simulink model "SimpleEKF_2007a"  (Simulink 6.6)
settings: Solver=FixedStepDiscrete  StartTime=0.0  StopTime=300  FixedStep=0.01  RelTol=1e-3
values from neighbouring files (symbols this model uses):
  initP = diag([ 1 1 1 1e5 1e5 1 1e5 1e5 1e5 ])    [SimpleEKF_init.m.m]
undefined symbols (not defined in the file or in its folder): DiscIntNeverNeededParam, gcbh, hwbcalib_subsystem
libraries: simulink x8, dspmtrx3 x5, dspinverses x1
(part 2 of 9)

== system SimpleEKF_2007a/EKF/skewSymmetric1 ==
  skewLibIn : Inport  OutDataType=fixdt(1,16,0)  OutScaling=[]
  column1 : Selector  Tag=MBDLibrary v2007b.1  IndexOptions=Index vector (dialog)  Indices=[7 3 5]  OutputSizes=1  InputPortWidth=7  mask(Mux Selector (MBDLibrary)){InputPortWidth_mbdlib=7, Indices_mbdlib=[7 3 5]}
      mask prompts: InputPortWidth_mbdlib "Input Port Width"; Indices_mbdlib "Output Indices"
      mask help: Changes the order of the inputs.
      settings: OpenFcn=|
      | if exist('mbdlib_dialog')
      |    mbdlib_dialog(gcb,'open')
      | else
      |    open_system(gcb, 'mask')
      | end
      settings: CloseFcn=|
      | if exist('mbdlib_selector')
      |    mbdlib_selector(gcb)
      | end
      mask Help: The SELECTOR block is a MULTIPLEXED SELECTOR block, used to change the input/output order of a multiplexed data stream.
      mask Display:
      | port_label('input', 1,'[7]')
      | text(1.0,0.83333,'7', 'horizontalAlignment', 'right')
      | text(1.0,0.5,'3', 'horizontalAlignment', 'right')
      | text(1.0,0.16667,'5', 'horizontalAlignment', 'right')
  column2 : Selector  Tag=MBDLibrary v2007b.1  IndexOptions=Index vector (dialog)  Indices=[6 7 1]  OutputSizes=1  InputPortWidth=7  mask(Mux Selector (MBDLibrary)){InputPortWidth_mbdlib=7, Indices_mbdlib=[6 7 1]}
      mask prompts: InputPortWidth_mbdlib "Input Port Width"; Indices_mbdlib "Output Indices"
      mask help: Changes the order of the inputs.
      settings: OpenFcn=|
      | if exist('mbdlib_dialog')
      |    mbdlib_dialog(gcb,'open')
      | else
      |    open_system(gcb, 'mask')
      | end
      settings: CloseFcn=|
      | if exist('mbdlib_selector')
      |    mbdlib_selector(gcb)
      | end
      mask Help: The SELECTOR block is a MULTIPLEXED SELECTOR block, used to change the input/output order of a multiplexed data stream.
      mask Display:
      | port_label('input', 1,'[7]')
      | text(1.0,0.83333,'6', 'horizontalAlignment', 'right')
      | text(1.0,0.5,'7', 'horizontalAlignment', 'right')
      | text(1.0,0.16667,'1', 'horizontalAlignment', 'right')
  column3 : Selector  Tag=MBDLibrary v2007b.1  IndexOptions=Index vector (dialog)  Indices=[2 4 7]  OutputSizes=1  InputPortWidth=7  mask(Mux Selector (MBDLibrary)){InputPortWidth_mbdlib=7, Indices_mbdlib=[2 4 7]}
      mask prompts: InputPortWidth_mbdlib "Input Port Width"; Indices_mbdlib "Output Indices"
      mask help: Changes the order of the inputs.
      settings: OpenFcn=|
      | if exist('mbdlib_dialog')
      |    mbdlib_dialog(gcb,'open')
      | else
      |    open_system(gcb, 'mask')
      | end
      settings: CloseFcn=|
      | if exist('mbdlib_selector')
      |    mbdlib_selector(gcb)
      | end
      mask Help: The SELECTOR block is a MULTIPLEXED SELECTOR block, used to change the input/output order of a multiplexed data stream.
      mask Display:
      | port_label('input', 1,'[7]')
      | text(1.0,0.83333,'2', 'horizontalAlignment', 'right')
      | text(1.0,0.5,'4', 'horizontalAlignment', 'right')
      | text(1.0,0.16667,'7', 'horizontalAlignment', 'right')
  matrixConcat : Concatenate  Tag=MBDLibrary v2007b.1  NumInputs=3  Mode=Multidimensional array  ConcatenateDimension=2  mask(Matrix Concat (MBDLibrary)){concatDim=Horizontal, numInputs_mbdlib=3}
      mask prompts: concatDim "Type of Concatenate"; numInputs_mbdlib "Number of Inputs"
      mask help: Concatenate input signals of the same data type to create a contiguous output signal.
      settings: OpenFcn=|
      | if exist('mbdlib_dialog')
      |    mbdlib_dialog(gcb,'open')
      | else
      |    open_system(gcb, 'mask')
      | end
      settings: CloseFcn=|
      | if exist('mbdlib_matrixConcatenate')
      |    mbdlib_matrixConcatenate(gcb, 'mask')
      | end
      mask Help:
      | The MATRIX CONCAT block concatenates input signals from the dame data type and creates a contigouos output matrix.
      | In vector mode, all input signals must be either vectors or one-row [1xM] matrices or one-column [Mx1] matrices or a combination of vectors and either one-row matrices or one-column matrices. The output is a vector if all inputs are vectors. The output is a one-row or one-column matrix if any of the inputs are one-row or one-column matrices respectively.
      | 
      | Matrix mode treats vector inputs as one-column matrices. The output is always a matrix.
      mask StyleString: popup(Vertical|Horizontal),edit
      mask Display:
      | plot([0.1 0.3 0.3 0.1 0.1], [0.1 0.1 0.9 0.9 0.1])
      | plot([0.4 0.6 0.6 0.4 0.4], [0.1 0.1 0.9 0.9 0.1])
      | plot([0.7 0.9 0.9 0.7 0.7], [0.1 0.1 0.9 0.9 0.1])
  mux : Mux  Tag=MBDLibrary v2007b.1  Inputs=3  mask(Mux (MBDLibrary)){Inputs_mbdlib=3}
      mask prompts: Inputs_mbdlib "Number of Inputs"
      mask help: Converts multipule inputs to a vector.
      settings: OpenFcn=|
      | if exist('mbdlib_dialog')
      |    mbdlib_dialog(gcb,'open')
      | else
      |    open_system(gcb, 'mask')
      | end
      mask Help: The MUX block provides a vector output to the model for separate inputs.  The output order will correspond to the input order (from the first input at the top of the block to the last input at the bottom of the block).
  negative : Gain  Tag=MBDLibrary v2007b.1  Gain=-1  ParameterDataType=fixdt(1,16,0)  ParameterScaling=[]  OutDataType=fixdt(1,16,0)  OutScaling=[]  RndMeth=Zero  mask(Gain (MBDLibrary)){gain_mbdlib=-1}
      mask prompts: gain_mbdlib "Gain"
      mask help: Multiplies the input by the gain.
      settings: OpenFcn=|
      | if exist('mbdlib_dialog')
      |    mbdlib_dialog(gcb,'open')
      | else
      |    open_system(gcb, 'mask')
      | end
      mask Help: The GAIN block multiplies the input by the gain value.  This block may accept any data types other than boolean.  The user must take care to not use a non-integer gain for int32/uint32 inputs.
      mask Display: disp([get_param(gcb, 'Gain') 'x'])
  zero : Constant  Tag=MBDLibrary v2007b.1  Value=0  VectorParams1D=off  OutDataType=fixdt(1,16,0)  OutScaling=[]  mask(Constant (MBDLibrary)){Value_mbdlib=0, OutDataTypeMode_mbdlib=double}
      mask prompts: Value_mbdlib "Constant"; OutDataTypeMode_mbdlib "Data Type"
      mask help: Outputs a constant value
      settings: AttributesFormatString={%<OutDataTypeMode>}
      settings: OpenFcn=|
      | if exist('mbdlib_dialog')
      |    mbdlib_dialog(gcb,'open')
      | else
      |    open_system(gcb, 'mask')
      | end
      settings: CloseFcn=|
      | if exist('mbdlib_dialog')
      |    mbdlib_constant(gcb)
      | end
      mask Help: The CONSTANT block outputs a constant value to the system.
      mask StyleString: edit,popup(double|single|boolean|int32|uint32)
  skewLibOut : Outport  OutDataType=fixdt(1,16,0)  OutScaling=[]
  wires:
  zero/1 -> mux/3
  negative/1 -> mux/2
  column3/1 -> matrixConcat/3
  column2/1 -> matrixConcat/2
  column1/1 -> matrixConcat/1
  matrixConcat/1 -> skewLibOut/1
  mux/1 -> column1/1, column3/1, column2/1
  skewLibIn/1 -> mux/1, negative/1

== system SimpleEKF_2007a/INS/Attitude update ==
  wBodyToEciInBody : Inport  OutDataType=fixdt(1,16,0)  OutScaling=[]
  wNavToEciInNav : Inport  Port=2  PortDimensions=3  SampleTime=0.01  OutDataType=fixdt(1,16,0)  OutScaling=[]
  reset : Inport  Port=3  PortDimensions=1  SampleTime=0.01  OutDataType=fixdt(1,16,0)  OutScaling=[]
  initCon : Inport  Port=4  SampleTime=0.01  OutDataType=fixdt(1,16,0)  OutScaling=[]
  Stage1 : Subsystem
  Stage2 : Subsystem
  dcmBodyToNav : Outport  OutDataType=fixdt(1,16,0)  OutScaling=[]
  att : Outport  Port=2  OutDataType=fixdt(1,16,0)  OutScaling=[]
  wires:
  wBodyToEciInBody/1 -> Stage1/1(wBodyToEciInBody), [wBodyToEciInBody]
  wNavToEciInNav/1 -> Stage1/2(wNavToEciInNav), [wNavToEciInNav]
  Stage1/1(dcmNavToBody(k-1)) -> Stage2/1(dcmNavToBody)
  [wBodyToEciInBody] -> Stage2/4(wBodyToEciInBody)
  [wNavToEciInNav] -> Stage2/5(wNavToEciInNav)
  Stage2/1(att) -> att/1
  reset/1 -> Stage2/3(reset), Stage1/3(reset)
  initCon/1 -> Stage2/2(initCon), Stage1/4(initCon)
  Stage2/2(dcmBodyToNav(k)) -> dcmBodyToNav/1

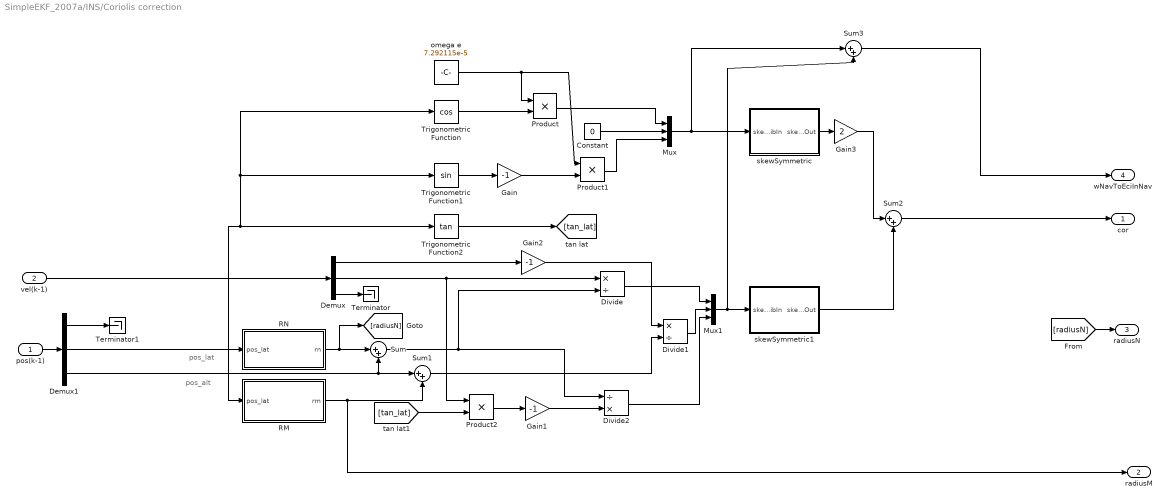
== system SimpleEKF_2007a/INS/Coriolis correction ==
  note: pos_alt
  note: pos_lat
  pos(k-1) : Inport  PortDimensions=3  SampleTime=0.01  OutDataType=fixdt(1,16,0)  OutScaling=[]
  vel(k-1) : Inport  Port=2  PortDimensions=3  SampleTime=0.01  OutDataType=fixdt(1,16,0)  OutScaling=[]
  Constant : Constant  Value=0  OutDataType=fixdt(1,16,0)  OutScaling=[]
  Demux : Demux  Outputs=3
  Demux1 : Demux  Outputs=3
  Divide : Product  Inputs=*/  OutDataType=fixdt(1,16,0)  OutScaling=[]
  Divide1 : Product  Inputs=*/  OutDataType=fixdt(1,16,0)  OutScaling=[]
  Divide2 : Product  Inputs=/*  OutDataType=fixdt(1,16,0)  OutScaling=[]  SampleTime=0.01
  Gain : Gain  Gain=-1  ParameterDataType=fixdt(1,16,0)  ParameterScaling=[]  OutDataType=fixdt(1,16,0)  OutScaling=[]
  Gain1 : Gain  Gain=-1  ParameterDataType=fixdt(1,16,0)  ParameterScaling=[]  OutDataType=fixdt(1,16,0)  OutScaling=[]
  Gain2 : Gain  Gain=-1  ParameterDataType=fixdt(1,16,0)  ParameterScaling=[]  OutDataType=fixdt(1,16,0)  OutScaling=[]
  Gain3 : Gain  Gain=2  ParameterDataType=fixdt(1,16,0)  ParameterScaling=[]  OutDataType=fixdt(1,16,0)  OutScaling=[]
  Mux : Mux  Inputs=3
  Mux1 : Mux  Inputs=3
  Product : Product  OutDataType=fixdt(1,16,0)  OutScaling=[]  RndMeth=Zero
  Product1 : Product  OutDataType=fixdt(1,16,0)  OutScaling=[]  RndMeth=Zero
  Product2 : Product  OutDataType=fixdt(1,16,0)  OutScaling=[]  RndMeth=Zero
  RM : Subsystem
  RN : Subsystem
  Sum : Sum  Inputs=|++  OutDataType=fixdt(1,16,0)  OutScaling=[]
  Sum1 : Sum  Inputs=|++  OutDataType=fixdt(1,16,0)  OutScaling=[]  SampleTime=0.01
  Sum2 : Sum  Inputs=|++  OutDataType=fixdt(1,16,0)  OutScaling=[]
  Sum3 : Sum  Inputs=|++  OutDataType=fixdt(1,16,0)  OutScaling=[]  SampleTime=0.01
  Terminator : Terminator
  Terminator1 : Terminator
  Trigonometric Function : Trigonometry  Operator=cos
  Trigonometric Function1 : Trigonometry
  Trigonometric Function2 : Trigonometry  Operator=tan
  omega e : Constant  Value=7.292115e-5  OutDataType=fixdt(1,16,0)  OutScaling=[]  SampleTime=0.01
  skewSymmetric : Subsystem  Tag=MBDLibrary v2007b.1  Description=|  TreatAsAtomicUnit=on
      | Skew Symmetric (MBDLibrary)                                                
      | Computes the Skew Symmetric Matrix Form of a vector.                       
      | output = [0  -omegaz omegay; omegaz 0 -omegax; -omegay omegax 0]           
      |                                                                            
      | %**************************************************************************
      | % HONEYWELL -CONFIDENTIAL: This copyrighted work and all information       
      | % are the property of Honeywell, contain trade secrets and may not,        
      | % in whole or in part, be used, duplicated, or disclosed for any purpose   
      | % without prior written permission of Honeywell.  All Rights Reserved.     
      | %                                                                          
      | % Notice                                                                   
      | % Freedom of Information Act (5 USC 552) and Disclosure of Confidential    
      | % Information Generally (18 USC 1905).  This material is being furnished   
      | % in confidence by Honeywell.  The information disclosed here falls        
      | % within exemption (b)(4) of 5 USC 552 and the prohibitions of             
      | % 18 USC 1905.                                                             
      | %                                                                          
      | % U.S. EXPORT CONTROL NOTICE:                                              
      | % This software is controlled in accordance with the United States Export  
      | % Administration Regulations (EAR).  This software has been classified as  
      | % EAR 99.  Diversion contrary to U.S. law is prohibited.                   
      | %**************************************************************************
      settings: OpenFcn=|
      | if exist('mbdlib_dialog')
      |    mbdlib_dialog(gcb,'open')
      | else
      |    open_system(gcb, 'mask')
      | end
      mask Type: Skew Symmetric (MBDLibrary)
      mask Description: Compute the Skew Symmetric Matrix Form of a Vector
      mask Help: The SKEW SYMMETRIC block computes the Skew Symmetric Matrix Form of a Vector
      mask Display:
      | plot([0.2 0.1 0.1 0.2], [0.95 0.95 0.05 0.05])
      | plot([0.8 0.9 0.9 0.8], [0.95 0.95 0.05 0.05])
      | text(0.5, 0.78, ' 0    -\omega_z   \omega_y', 'texmode', 'on')
      | text(0.5, 0.5, '  \omega_z   0   -\omega_x', 'texmode', 'on')
      | text(0.5, 0.22, '-\omega_y   \omega_x   0', 'texmode', 'on')
  skewSymmetric1 : Subsystem  Tag=MBDLibrary v2007b.1  Description=|  TreatAsAtomicUnit=on
      | Skew Symmetric (MBDLibrary)                                                
      | Computes the Skew Symmetric Matrix Form of a vector.                       
      | output = [0  -omegaz omegay; omegaz 0 -omegax; -omegay omegax 0]           
      |                                                                            
      | %**************************************************************************
      | % HONEYWELL -CONFIDENTIAL: This copyrighted work and all information       
      | % are the property of Honeywell, contain trade secrets and may not,        
      | % in whole or in part, be used, duplicated, or disclosed for any purpose   
      | % without prior written permission of Honeywell.  All Rights Reserved.     
      | %                                                                          
      | % Notice                                                                   
      | % Freedom of Information Act (5 USC 552) and Disclosure of Confidential    
      | % Information Generally (18 USC 1905).  This material is being furnished   
      | % in confidence by Honeywell.  The information disclosed here falls        
      | % within exemption (b)(4) of 5 USC 552 and the prohibitions of             
      | % 18 USC 1905.                                                             
      | %                                                                          
      | % U.S. EXPORT CONTROL NOTICE:                                              
      | % This software is controlled in accordance with the United States Export  
      | % Administration Regulations (EAR).  This software has been classified as  
      | % EAR 99.  Diversion contrary to U.S. law is prohibited.                   
      | %**************************************************************************
      settings: OpenFcn=|
      | if exist('mbdlib_dialog')
      |    mbdlib_dialog(gcb,'open')
      | else
      |    open_system(gcb, 'mask')
      | end
      mask Type: Skew Symmetric (MBDLibrary)
      mask Description: Compute the Skew Symmetric Matrix Form of a Vector
      mask Help: The SKEW SYMMETRIC block computes the Skew Symmetric Matrix Form of a Vector
      mask Display:
      | plot([0.2 0.1 0.1 0.2], [0.95 0.95 0.05 0.05])
      | plot([0.8 0.9 0.9 0.8], [0.95 0.95 0.05 0.05])
      | text(0.5, 0.78, ' 0    -\omega_z   \omega_y', 'texmode', 'on')
      | text(0.5, 0.5, '  \omega_z   0   -\omega_x', 'texmode', 'on')
      | text(0.5, 0.22, '-\omega_y   \omega_x   0', 'texmode', 'on')
  cor : Outport  PortDimensions=[3,3]  SampleTime=0.01  OutDataType=fixdt(1,16,0)  OutScaling=[]
  radiusM : Outport  Port=2  OutDataType=fixdt(1,16,0)  OutScaling=[]
  radiusN : Outport  Port=3  OutDataType=fixdt(1,16,0)  OutScaling=[]
  wNavToEciInNav : Outport  Port=4  PortDimensions=3  SampleTime=0.01  OutDataType=fixdt(1,16,0)  OutScaling=[]
  wires:
  vel(k-1)/1 -> Demux/1
  omega e/1 -> Product/1, Product1/1
  Trigonometric Function/1 -> Product/2
  Trigonometric Function1/1 -> Gain/1
  Gain/1 -> Product1/2
  Product/1 -> Mux/1
  Constant/1 -> Mux/2
  Product1/1 -> Mux/3
  RN/1(rn) -> Sum/1, [radiusN]
  Demux/2 -> Product2/1, Divide/1
  Product2/1 -> Gain1/1
  Sum/1 -> Divide/2, Divide2/1
  Demux/1 -> Gain2/1
  Gain2/1 -> Divide1/1
  Sum1/1 -> Divide1/2
  Divide/1 -> Mux1/1
  Divide1/1 -> Mux1/2
  Mux1/1 -> skewSymmetric1/1(skewLibIn), Sum3/2
  skewSymmetric/1(skewLibOut) -> Gain3/1
  Gain3/1 -> Sum2/1
  skewSymmetric1/1(skewLibOut) -> Sum2/2
  pos(k-1)/1 -> Demux1/1
  Demux/3 -> Terminator/1
  RM/1(rm) -> Sum1/2, radiusM/1
  Demux1/3 -> Sum1/1, Sum/2
  Demux1/1 -> Terminator1/1
  Sum2/1 -> cor/1
  Mux/1 -> skewSymmetric/1(skewLibIn), Sum3/1
  Demux1/2 -> RM/1(pos_lat), Trigonometric Function2/1, Trigonometric Function/1, Trigonometric Function1/1, RN/1(pos_lat)
  Sum3/1 -> wNavToEciInNav/1
  [radiusN] -> radiusN/1
  Gain1/1 -> Divide2/2
  [tan_lat] -> Product2/2
  Trigonometric Function2/1 -> [tan_lat]
  Divide2/1 -> Mux1/3

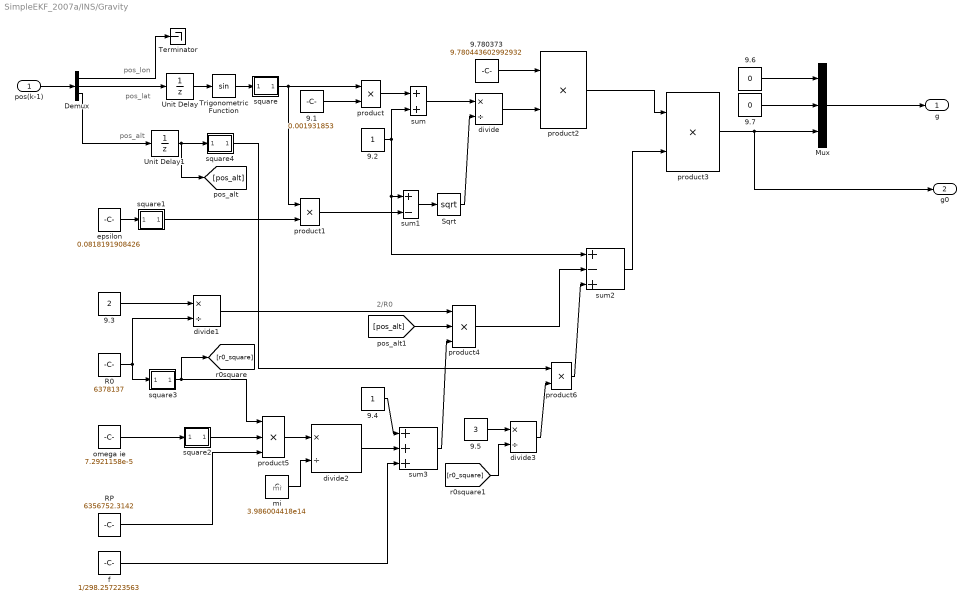
== system SimpleEKF_2007a/INS/Gravity ==
  note: pos_lat
  note: pos_alt
  note: 2/R0
  note: pos_lon
  note: mi
  pos(k-1) : Inport  PortDimensions=3  SampleTime=0.01  OutDataType=fixdt(1,16,0)  OutScaling=[]
  9.1 : Constant  Value=0.001931853  OutDataTypeMode=double  OutDataType=fixdt(1,16,0)  OutScaling=[]
  9.2 : Constant  OutDataTypeMode=double  OutDataType=fixdt(1,16,0)  OutScaling=[]
  9.3 : Constant  Value=2  OutDataTypeMode=double  OutDataType=fixdt(1,16,0)  OutScaling=[]
  9.4 : Constant  OutDataTypeMode=double  OutDataType=fixdt(1,16,0)  OutScaling=[]
  9.5 : Constant  Value=3  OutDataTypeMode=double  OutDataType=fixdt(1,16,0)  OutScaling=[]
  9.6 : Constant  Value=0  OutDataTypeMode=double  OutDataType=fixdt(1,16,0)  OutScaling=[]
  9.7 : Constant  Value=0  OutDataTypeMode=double  OutDataType=fixdt(1,16,0)  OutScaling=[]
  9.780373 : Constant  Value=9.780443602992932  OutDataTypeMode=double  OutDataType=fixdt(1,16,0)  OutScaling=[]  SampleTime=0.01
  Demux : Demux  Outputs=3
  Mux : Mux  Inputs=3
  R0 : Constant  Value=6378137  OutDataType=fixdt(1,16,0)  OutScaling=[]
  RP : Constant  Value=6356752.3142  OutDataType=fixdt(1,16,0)  OutScaling=[]
  Sqrt : Math  Operator=sqrt  OutDataType=fixdt(1,16,0)  OutScaling=[]  SaturateOnIntegerOverflow=on
  Terminator : Terminator
  Trigonometric Function : Trigonometry
  Unit Delay : UnitDelay  X0=0.7853981633974483  SampleTime=0.01
  Unit Delay1 : UnitDelay  X0=0.7853981633974483  SampleTime=0.01
  divide{,1..3} (4 alike) : Product  Tag=MBDLibrary v2007b.1  Inputs=*/  OutDataType=fixdt(1,16,0)  OutScaling=[]  RndMeth=Zero  InputSameDT=on
      settings: OpenFcn=|
      | if exist('mbdlib_dialog')
      |    mbdlib_dialog(gcb,'open')
      | else
      |    open_system(gcb, 'mask')
      | end
      mask Type: Divide (MBDLibrary)
      mask Description: Divides two inputs.
      mask Help: file:///c:\Program Files\MATLAB\R2007b\toolbox\Guidance_and_Navigation_Global\help_files\GeneralUtilities\MBDLibrary\mathfunctions\divide.html
      mask Display:
      | port_label('input',1,'n')
      | port_label('input',2,'d')
      | port_label('output',1,'n/d')
  epsilon : Constant  Value=0.0818191908426  OutDataType=fixdt(1,16,0)  OutScaling=[]
  f : Constant  Value=1/298.257223563  OutDataType=fixdt(1,16,0)  OutScaling=[]
  mi : Constant  Value=3.986004418e14  OutDataType=fixdt(1,16,0)  OutScaling=[]
  omega ie : Constant  Value=7.2921158e-5  OutDataType=fixdt(1,16,0)  OutScaling=[]
  product : Product  Tag=MBDLibrary v2007b.1  OutDataType=fixdt(1,16,0)  OutScaling=[]  RndMeth=Zero  InputSameDT=on  mask(Product (MBDLibrary)){Inputs_mbdlib=2}
      mask prompts: Inputs_mbdlib "Number of Inputs"
      mask help: Multiplies inputs.
      settings: OpenFcn=|
      | if exist('mbdlib_dialog')
      |    mbdlib_dialog(gcb,'open')
      | else
      |    open_system(gcb, 'mask')
      | end
      mask Help: file:///c:\Program Files\MATLAB\R2007b\toolbox\Guidance_and_Navigation_Global\help_files\GeneralUtilities\MBDLibrary\mathfunctions\product.html
  product1 : Product  Tag=MBDLibrary v2007b.1  OutDataType=fixdt(1,16,0)  OutScaling=[]  RndMeth=Zero  InputSameDT=on  mask(Product (MBDLibrary)){Inputs_mbdlib=2}
      mask prompts: Inputs_mbdlib "Number of Inputs"
      mask help: Multiplies inputs.
      settings: OpenFcn=|
      | if exist('mbdlib_dialog')
      |    mbdlib_dialog(gcb,'open')
      | else
      |    open_system(gcb, 'mask')
      | end
      mask Help: file:///c:\Program Files\MATLAB\R2007b\toolbox\Guidance_and_Navigation_Global\help_files\GeneralUtilities\MBDLibrary\mathfunctions\product.html
  product2 : Product  Tag=MBDLibrary v2007b.1  OutDataType=fixdt(1,16,0)  OutScaling=[]  RndMeth=Zero  InputSameDT=on  mask(Product (MBDLibrary)){Inputs_mbdlib=2}
      mask prompts: Inputs_mbdlib "Number of Inputs"
      mask help: Multiplies inputs.
      settings: OpenFcn=|
      | if exist('mbdlib_dialog')
      |    mbdlib_dialog(gcb,'open')
      | else
      |    open_system(gcb, 'mask')
      | end
      mask Help: file:///c:\Program Files\MATLAB\R2007b\toolbox\Guidance_and_Navigation_Global\help_files\GeneralUtilities\MBDLibrary\mathfunctions\product.html
  product3 : Product  Tag=MBDLibrary v2007b.1  OutDataType=fixdt(1,16,0)  OutScaling=[]  RndMeth=Zero  InputSameDT=on  mask(Product (MBDLibrary)){Inputs_mbdlib=2}
      mask prompts: Inputs_mbdlib "Number of Inputs"
      mask help: Multiplies inputs.
      settings: OpenFcn=|
      | if exist('mbdlib_dialog')
      |    mbdlib_dialog(gcb,'open')
      | else
      |    open_system(gcb, 'mask')
      | end
      mask Help: file:///c:\Program Files\MATLAB\R2007b\toolbox\Guidance_and_Navigation_Global\help_files\GeneralUtilities\MBDLibrary\mathfunctions\product.html
  product4 : Product  Tag=MBDLibrary v2007b.1  Inputs=3  OutDataType=fixdt(1,16,0)  OutScaling=[]  RndMeth=Zero  InputSameDT=on  mask(Product (MBDLibrary)){Inputs_mbdlib=3}
      mask prompts: Inputs_mbdlib "Number of Inputs"
      mask help: Multiplies inputs.
      settings: OpenFcn=|
      | if exist('mbdlib_dialog')
      |    mbdlib_dialog(gcb,'open')
      | else
      |    open_system(gcb, 'mask')
      | end
      mask Help: file:///c:\Program Files\MATLAB\R2007b\toolbox\Guidance_and_Navigation_Global\help_files\GeneralUtilities\MBDLibrary\mathfunctions\product.html
  product5 : Product  Tag=MBDLibrary v2007b.1  Inputs=3  OutDataType=fixdt(1,16,0)  OutScaling=[]  RndMeth=Zero  InputSameDT=on  mask(Product (MBDLibrary)){Inputs_mbdlib=3}
      mask prompts: Inputs_mbdlib "Number of Inputs"
      mask help: Multiplies inputs.
      settings: OpenFcn=|
      | if exist('mbdlib_dialog')
      |    mbdlib_dialog(gcb,'open')
      | else
      |    open_system(gcb, 'mask')
      | end
      mask Help: file:///c:\Program Files\MATLAB\R2007b\toolbox\Guidance_and_Navigation_Global\help_files\GeneralUtilities\MBDLibrary\mathfunctions\product.html
  product6 : Product  Tag=MBDLibrary v2007b.1  OutDataType=fixdt(1,16,0)  OutScaling=[]  RndMeth=Zero  InputSameDT=on  mask(Product (MBDLibrary)){Inputs_mbdlib=2}
      mask prompts: Inputs_mbdlib "Number of Inputs"
      mask help: Multiplies inputs.
      settings: OpenFcn=|
      | if exist('mbdlib_dialog')
      |    mbdlib_dialog(gcb,'open')
      | else
      |    open_system(gcb, 'mask')
      | end
      mask Help: file:///c:\Program Files\MATLAB\R2007b\toolbox\Guidance_and_Navigation_Global\help_files\GeneralUtilities\MBDLibrary\mathfunctions\product.html
  square : Subsystem  Tag=MBDLibrary v2007b.1
      settings: OpenFcn=|
      | if exist('mbdlib_dialog')
      |    mbdlib_dialog(gcb,'open')
      | else
      |    open_system(gcb, 'mask')
      | end
      mask Type: Square (MBDLibrary)
      mask Description: Squares the input.
      mask Help: file:///c:\Program Files\MATLAB\R2007b\toolbox\Guidance_and_Navigation_Global\help_files\GeneralUtilities\MBDLibrary\mathfunctions\square.html
      mask Display: disp('x^2', 'texmode', 'on')
  square1 : Subsystem  Tag=MBDLibrary v2007b.1
      settings: OpenFcn=|
      | if exist('mbdlib_dialog')
      |    mbdlib_dialog(gcb,'open')
      | else
      |    open_system(gcb, 'mask')
      | end
      mask Type: Square (MBDLibrary)
      mask Description: Squares the input.
      mask Help: file:///c:\Program Files\MATLAB\R2007b\toolbox\Guidance_and_Navigation_Global\help_files\GeneralUtilities\MBDLibrary\mathfunctions\square.html
      mask Display: disp('x^2', 'texmode', 'on')
  square2 : Subsystem  Tag=MBDLibrary v2007b.1
      settings: OpenFcn=|
      | if exist('mbdlib_dialog')
      |    mbdlib_dialog(gcb,'open')
      | else
      |    open_system(gcb, 'mask')
      | end
      mask Type: Square (MBDLibrary)
      mask Description: Squares the input.
      mask Help: file:///c:\Program Files\MATLAB\R2007b\toolbox\Guidance_and_Navigation_Global\help_files\GeneralUtilities\MBDLibrary\mathfunctions\square.html
      mask Display: disp('x^2', 'texmode', 'on')
  square3 : Subsystem  Tag=MBDLibrary v2007b.1
      settings: OpenFcn=|
      | if exist('mbdlib_dialog')
      |    mbdlib_dialog(gcb,'open')
      | else
      |    open_system(gcb, 'mask')
      | end
      mask Type: Square (MBDLibrary)
      mask Description: Squares the input.
      mask Help: file:///c:\Program Files\MATLAB\R2007b\toolbox\Guidance_and_Navigation_Global\help_files\GeneralUtilities\MBDLibrary\mathfunctions\square.html
      mask Display: disp('x^2', 'texmode', 'on')
  square4 : Subsystem  Tag=MBDLibrary v2007b.1
      settings: OpenFcn=|
      | if exist('mbdlib_dialog')
      |    mbdlib_dialog(gcb,'open')
      | else
      |    open_system(gcb, 'mask')
      | end
      mask Type: Square (MBDLibrary)
      mask Description: Squares the input.
      mask Help: file:///c:\Program Files\MATLAB\R2007b\toolbox\Guidance_and_Navigation_Global\help_files\GeneralUtilities\MBDLibrary\mathfunctions\square.html
      mask Display: disp('x^2', 'texmode', 'on')
  sum : Sum  Tag=MBDLibrary v2007b.1  OutDataType=fixdt(1,16,0)  OutScaling=[]  RndMeth=Zero  InputSameDT=on  mask(Sum (MBDLibrary)){inputs_mbdlib=++}
      mask prompts: inputs_mbdlib "List of signs"
      mask help: Adds values together.
      settings: OpenFcn=|
      | if exist('mbdlib_dialog')
      |    mbdlib_dialog(gcb,'open')
      | else
      |    open_system(gcb, 'mask')
      | end
      mask Help: file:///c:\Program Files\MATLAB\R2007b\toolbox\Guidance_and_Navigation_Global\help_files\GeneralUtilities\MBDLibrary\mathfunctions\sum.html
  sum1 : Sum  Tag=MBDLibrary v2007b.1  Inputs=+-  OutDataType=fixdt(1,16,0)  OutScaling=[]  RndMeth=Zero  InputSameDT=on  mask(Sum (MBDLibrary)){inputs_mbdlib=+-}
      mask prompts: inputs_mbdlib "List of signs"
      mask help: Adds values together.
      settings: OpenFcn=|
      | if exist('mbdlib_dialog')
      |    mbdlib_dialog(gcb,'open')
      | else
      |    open_system(gcb, 'mask')
      | end
      mask Help: file:///c:\Program Files\MATLAB\R2007b\toolbox\Guidance_and_Navigation_Global\help_files\GeneralUtilities\MBDLibrary\mathfunctions\sum.html
  sum2 : Sum  Tag=MBDLibrary v2007b.1  Inputs=+-+  OutDataType=fixdt(1,16,0)  OutScaling=[]  RndMeth=Zero  InputSameDT=on  mask(Sum (MBDLibrary)){inputs_mbdlib=+-+}
      mask prompts: inputs_mbdlib "List of signs"
      mask help: Adds values together.
      settings: OpenFcn=|
      | if exist('mbdlib_dialog')
      |    mbdlib_dialog(gcb,'open')
      | else
      |    open_system(gcb, 'mask')
      | end
      mask Help: file:///c:\Program Files\MATLAB\R2007b\toolbox\Guidance_and_Navigation_Global\help_files\GeneralUtilities\MBDLibrary\mathfunctions\sum.html
  sum3 : Sum  Tag=MBDLibrary v2007b.1  Inputs=+++  OutDataType=fixdt(1,16,0)  OutScaling=[]  RndMeth=Zero  InputSameDT=on  mask(Sum (MBDLibrary)){inputs_mbdlib=+++}
      mask prompts: inputs_mbdlib "List of signs"
      mask help: Adds values together.
      settings: OpenFcn=|
      | if exist('mbdlib_dialog')
      |    mbdlib_dialog(gcb,'open')
      | else
      |    open_system(gcb, 'mask')
      | end
      mask Help: file:///c:\Program Files\MATLAB\R2007b\toolbox\Guidance_and_Navigation_Global\help_files\GeneralUtilities\MBDLibrary\mathfunctions\sum.html
  g : Outport  PortDimensions=3  SampleTime=0.01  OutDataType=fixdt(1,16,0)  OutScaling=[]
  g0 : Outport  Port=2  PortDimensions=1  SampleTime=0.01  OutDataType=fixdt(1,16,0)  OutScaling=[]
  wires:
  9.6/1 -> Mux/1
  9.7/1 -> Mux/2
  Mux/1 -> g/1
  Demux/1 -> Terminator/1
  pos(k-1)/1 -> Demux/1
  Demux/2 -> Unit Delay/1
  Trigonometric Function/1 -> square/1(squareLibIn)
  9.1/1 -> product/2
  product/1 -> sum/1
  9.2/1 -> sum/2, sum1/1, sum2/1
  sum/1 -> divide/1
  epsilon/1 -> square1/1(squareLibIn)
  square1/1(squareLibOut) -> product1/2
  product1/1 -> sum1/2
  sum1/1 -> Sqrt/1
  Sqrt/1 -> divide/2
  9.780373/1 -> product2/1
  divide/1 -> product2/2
  product2/1 -> product3/1
  9.3/1 -> divide1/1
  R0/1 -> divide1/2, square3/1(squareLibIn)
  divide1/1 -> product4/1
  9.4/1 -> sum3/1
  omega ie/1 -> square2/1(squareLibIn)
  square3/1(squareLibOut) -> product5/1, [r0_square]
  square2/1(squareLibOut) -> product5/2
  RP/1 -> product5/3
  product5/1 -> divide2/1
  mi/1 -> divide2/2
  product4/1 -> sum2/2
  9.5/1 -> divide3/1
  Demux/3 -> Unit Delay1/1
  square4/1(squareLibOut) -> product6/1
  product3/1 -> Mux/3, g0/1
  Unit Delay/1 -> Trigonometric Function/1
  divide3/1 -> product6/2
  product6/1 -> sum2/3
  sum2/1 -> product3/2
  [pos_alt] -> product4/2
  sum3/1 -> product4/3
  divide2/1 -> sum3/2
  f/1 -> sum3/3
  [r0_square] -> divide3/2
  square/1(squareLibOut) -> product/1, product1/1
  Unit Delay1/1 -> square4/1(squareLibIn), [pos_alt]

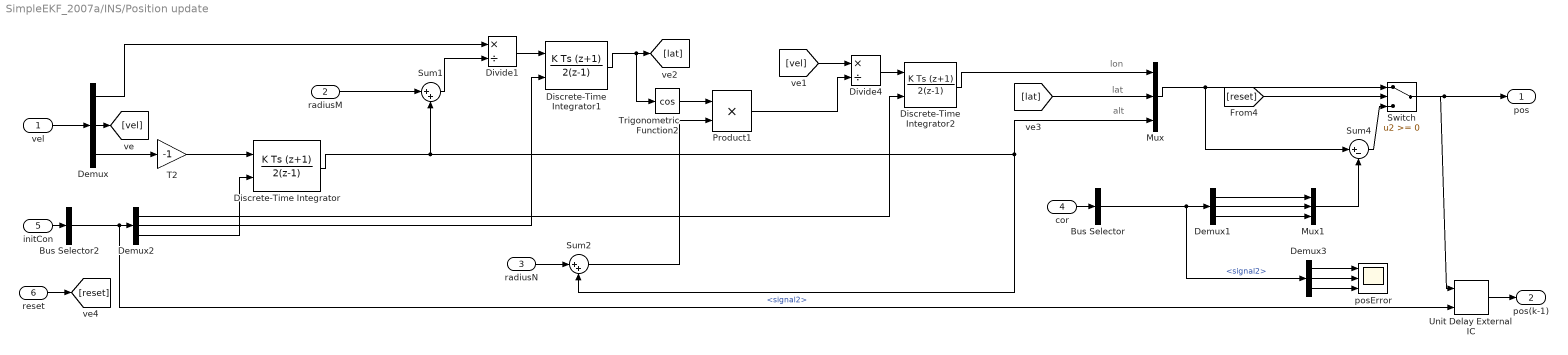
== system SimpleEKF_2007a/INS/Position update ==
  note: alt
  note: lat
  note: lon
  vel : Inport  PortDimensions=3  SampleTime=0.01  OutDataType=fixdt(1,16,0)  OutScaling=[]
  radiusM : Inport  Port=2  PortDimensions=1  SampleTime=0.01  OutDataType=fixdt(1,16,0)  OutScaling=[]
  radiusN : Inport  Port=3  PortDimensions=1  SampleTime=0.01  OutDataType=fixdt(1,16,0)  OutScaling=[]
  cor : Inport  Port=4  OutDataType=fixdt(1,16,0)  OutScaling=[]
  initCon : Inport  Port=5  OutDataType=fixdt(1,16,0)  OutScaling=[]
  reset : Inport  Port=6  OutDataType=fixdt(1,16,0)  OutScaling=[]
  Bus Selector : BusSelector  OutputSignals=signal2
  Bus Selector2 : BusSelector  OutputSignals=signal2
  Demux{,1..3} (4 alike) : Demux  Outputs=3
  Discrete-Time Integrator : DiscreteIntegrator  IntegratorMethod=Integration: Trapezoidal  InitialConditionSource=external  SampleTime=0.01  OutDataType=fixdt(1,16,0)  OutScaling=[]  ICPrevOutput=DiscIntNeverNeededParam  ICPrevScaledInput=DiscIntNeverNeededParam
  Discrete-Time Integrator1 : DiscreteIntegrator  IntegratorMethod=Integration: Trapezoidal  InitialConditionSource=external  InitialCondition=0.7853981633974483  SampleTime=0.01  OutDataType=fixdt(1,16,0)  OutScaling=[]  ICPrevOutput=DiscIntNeverNeededParam  ICPrevScaledInput=DiscIntNeverNeededParam
  Discrete-Time Integrator2 : DiscreteIntegrator  IntegratorMethod=Integration: Trapezoidal  InitialConditionSource=external  InitialCondition=1.570796326794897  SampleTime=0.01  OutDataType=fixdt(1,16,0)  OutScaling=[]  ICPrevOutput=DiscIntNeverNeededParam  ICPrevScaledInput=DiscIntNeverNeededParam
  Divide1 : Product  Inputs=*/  OutDataType=fixdt(1,16,0)  OutScaling=[]
  Divide4 : Product  Inputs=*/  OutDataType=fixdt(1,16,0)  OutScaling=[]
  Mux : Mux  Inputs=3
  Mux1 : Mux  Inputs=3
  Product1 : Product  OutDataType=fixdt(1,16,0)  OutScaling=[]  RndMeth=Zero
  Sum1 : Sum  Inputs=|++  OutDataType=fixdt(1,16,0)  OutScaling=[]
  Sum2 : Sum  Inputs=|++  OutDataType=fixdt(1,16,0)  OutScaling=[]  SampleTime=0.01
  Sum4 : Sum  Inputs=|+-  OutDataType=fixdt(1,16,0)  OutScaling=[]
  Switch : Switch  SampleTime=0.01
  T2 : Gain  Gain=-1  ParameterDataType=fixdt(1,16,0)  ParameterScaling=[]  OutDataType=fixdt(1,16,0)  OutScaling=[]  SampleTime=0.01
  Trigonometric Function2 : Trigonometry  Operator=cos
  Unit Delay External IC : simulink/Additional Math & Discrete/Additional Discrete/Unit Delay External IC  SystemSampleTime=-1  tsamp=-1
  posError : Scope  NumInputPorts=3
      settings: TimeRange=100  YMin=2.25e-006~-2.5e-006~-13.5  YMax=4.25e-006~2.11758e-022~-7  SaveName=ScopeData12
  pos : Outport  OutDataType=fixdt(1,16,0)  OutScaling=[]
  pos(k-1) : Outport  Port=2  OutDataType=fixdt(1,16,0)  OutScaling=[]
  wires:
  Demux/1 -> Divide1/1
  vel/1 -> Demux/1
  Demux/3 -> T2/1
  T2/1 -> Discrete-Time Integrator/1
  Sum1/1 -> Divide1/2
  radiusM/1 -> Sum1/1
  Divide1/1 -> Discrete-Time Integrator1/1
  Discrete-Time Integrator1/1 -> Trigonometric Function2/1, [lat]
  radiusN/1 -> Sum2/1
  Trigonometric Function2/1 -> Product1/1
  Sum2/1 -> Product1/2
  Product1/1 -> Divide4/2
  Divide4/1 -> Discrete-Time Integrator2/1
  Discrete-Time Integrator2/1 -> Mux/1
  Demux/2 -> [vel]
  [vel] -> Divide4/1
  Discrete-Time Integrator/1 -> Mux/3, Sum2/2, Sum1/2
  [lat] -> Mux/2
  [reset] -> Switch/2
  Sum4/1 -> Switch/3
  cor/1 -> Bus Selector/1
  Mux/1 -> Switch/1, Sum4/1
  initCon/1 -> Bus Selector2/1
  Bus Selector2/1 -> Demux2/1, Unit Delay External IC/2  "<signal2>"
  Demux2/3 -> Discrete-Time Integrator/2
  Demux2/2 -> Discrete-Time Integrator1/2
  Demux2/1 -> Discrete-Time Integrator2/2
  reset/1 -> [reset]
  Switch/1 -> pos/1, Unit Delay External IC/1
  Unit Delay External IC/1 -> pos(k-1)/1
  Bus Selector/1 -> Demux1/1, Demux3/1  "<signal2>"
  Mux1/1 -> Sum4/2
  Demux3/1 -> posError/1
  Demux3/2 -> posError/2
  Demux3/3 -> posError/3
  Demux1/3 -> Mux1/3
  Demux1/1 -> Mux1/1
  Demux1/2 -> Mux1/2

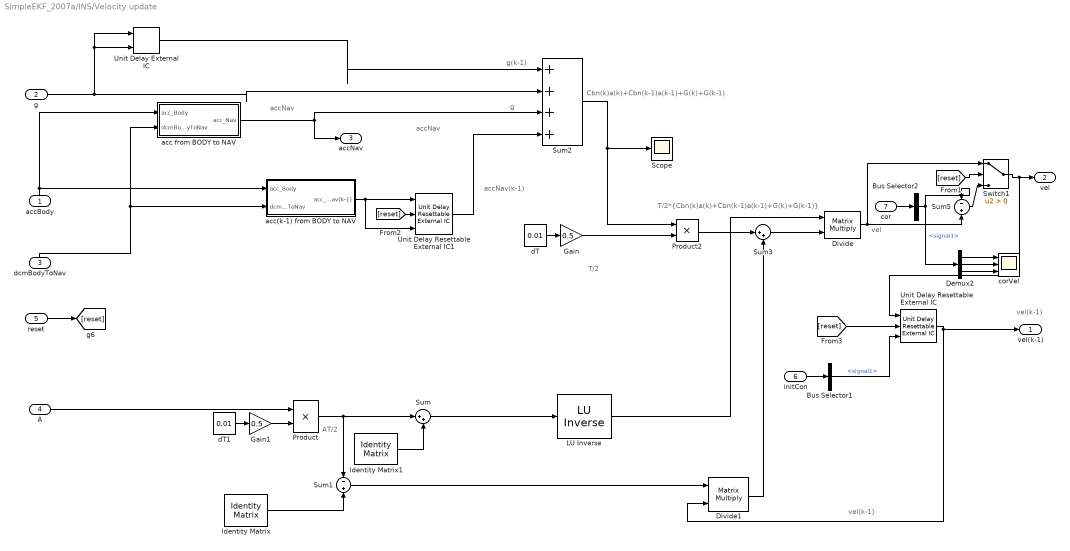
== system SimpleEKF_2007a/INS/Velocity update ==
  note: accNav
  note: g
  note: g(k-1)
  note: T/2*{Cbn(k)a(k)+Cbn(k-1)a(k-1)+G(k)+G(k-1)}
  note: Cbn(k)a(k)+Cbn(k-1)a(k-1)+G(k)+G(k-1)
  note: T/2
  note: vel
  note: accNav(k-1)
  note: vel(k-1)
  note: AT/2
  note: vel(k-1)
  note: accNav
  accBody : Inport  Orientation=up  PortDimensions=3  SampleTime=0.01  OutDataType=fixdt(1,16,0)  OutScaling=[]
  g : Inport  Port=2  PortDimensions=3  SampleTime=0.01  OutDataType=fixdt(1,16,0)  OutScaling=[]
  dcmBodyToNav : Inport  Orientation=up  Port=3  PortDimensions=[3,3]  SampleTime=0.01  OutDataType=fixdt(1,16,0)  OutScaling=[]
  A : Inport  Port=4  PortDimensions=[3,3]  SampleTime=0.01  OutDataType=fixdt(1,16,0)  OutScaling=[]
  reset : Inport  Port=5  PortDimensions=1  SampleTime=0.01  OutDataType=fixdt(1,16,0)  OutScaling=[]
  initCon : Inport  Port=6  OutDataType=fixdt(1,16,0)  OutScaling=[]
  cor : Inport  Port=7  OutDataType=fixdt(1,16,0)  OutScaling=[]
  " LU Inverse" : dspinverses/ LU Inverse  SystemSampleTime=-1
  Bus Selector1 : BusSelector  OutputSignals=signal1
  Bus Selector2 : BusSelector  OutputSignals=signal1
  Demux2 : Demux  Outputs=3
  Divide : Product  Inputs=**  Multiplication=Matrix(*)  OutDataType=fixdt(1,16,0)  OutScaling=[]  SampleTime=0.01
  Divide1 : Product  Inputs=**  Multiplication=Matrix(*)  OutDataType=fixdt(1,16,0)  OutScaling=[]  SampleTime=0.01
  Gain : Gain  Gain=0.5  ParameterDataType=fixdt(1,16,0)  ParameterScaling=[]  OutDataType=fixdt(1,16,0)  OutScaling=[]  SampleTime=0.01
  Gain1 : Gain  Gain=0.5  ParameterDataType=fixdt(1,16,0)  ParameterScaling=[]  OutDataType=fixdt(1,16,0)  OutScaling=[]  SampleTime=0.01
  Identity Matrix : dspmtrx3/Identity Matrix  Inherit=off  N=[3]  Ts=0.01  dataType=double  isSigned=on  wordLen=16  udDataType=sfix(16)  fracBitsMode=Best precision  numFracBits=15
  Identity Matrix1 : dspmtrx3/Identity Matrix  Inherit=off  N=[3]  Ts=0.01  dataType=double  isSigned=on  wordLen=16  udDataType=sfix(16)  fracBitsMode=Best precision  numFracBits=15
  Product : Product  OutDataType=fixdt(1,16,0)  OutScaling=[]  RndMeth=Zero
  Product2 : Product  OutDataType=fixdt(1,16,0)  OutScaling=[]  SampleTime=0.01  RndMeth=Zero
  Scope : Scope
      settings: SaveName=ScopeData11
  Sum : Sum  Inputs=|++  OutDataType=fixdt(1,16,0)  OutScaling=[]  SampleTime=0.01
  Sum1 : Sum  Inputs=-+  OutDataType=fixdt(1,16,0)  OutScaling=[]
  Sum2 : Sum  Inputs=|++++  OutDataType=fixdt(1,16,0)  OutScaling=[]  SampleTime=0.01
  Sum3 : Sum  Inputs=|++  OutDataType=fixdt(1,16,0)  OutScaling=[]  SampleTime=0.01
  Sum5 : Sum  Inputs=-+  OutDataType=fixdt(1,16,0)  OutScaling=[]
  Switch1 : Switch  Criteria=u2 > Threshold  SampleTime=0.01
  Unit Delay External IC : simulink/Additional Math & Discrete/Additional Discrete/Unit Delay External IC  SystemSampleTime=-1  tsamp=-1
  Unit Delay Resettable External IC : simulink/Additional Math & Discrete/Additional Discrete/Unit Delay Resettable External IC  SystemSampleTime=-1  tsamp=0.01
  Unit Delay Resettable External IC1 : simulink/Additional Math & Discrete/Additional Discrete/Unit Delay Resettable External IC  SystemSampleTime=-1  tsamp=-1
  acc from BODY to NAV : Subsystem
  acc(k-1) from BODY to NAV : Subsystem
  corVel : Scope  NumInputPorts=3
      settings: TimeRange=300  YMin=-25.5~-3.3~-21.5  YMax=-19~-2.75~-16  SaveName=ScopeData8
  dT : Constant  Value=0.01  OutDataType=fixdt(1,16,0)  OutScaling=[]  SampleTime=0.01
  dT1 : Constant  Value=0.01  OutDataType=fixdt(1,16,0)  OutScaling=[]  SampleTime=0.01
  vel(k-1) : Outport  PortDimensions=3  SampleTime=0.01  OutDataType=fixdt(1,16,0)  OutScaling=[]
  vel : Outport  Port=2  PortDimensions=3  SampleTime=0.01  OutDataType=fixdt(1,16,0)  OutScaling=[]
  accNav : Outport  Port=3  PortDimensions=3  SampleTime=0.01  OutDataType=fixdt(1,16,0)  OutScaling=[]
  wires:
  Sum2/1 -> Product2/1, Scope/1
  Product2/1 -> Sum3/1
  dT/1 -> Gain/1
  Sum3/1 -> Divide/2
  accBody/1 -> acc from BODY to NAV/1(acc_Body), acc(k-1) from BODY to NAV/1(acc_Body)
  dcmBodyToNav/1 -> acc from BODY to NAV/2(dcmBodyToNav), acc(k-1) from BODY to NAV/2(dcmBodyToNav)
  Divide/1 -> Sum5/2, Switch1/1
  A/1 -> Product/1
  Gain/1 -> Product2/2
  g/1 -> Sum2/2, Unit Delay External IC/1, Unit Delay External IC/2
  acc from BODY to NAV/1(acc_Nav) -> Sum2/3, accNav/1
  Product/1 -> Sum/1, Sum1/1
  Sum/1 -> " LU Inverse"/1
  Identity Matrix/1 -> Sum1/2
  " LU Inverse"/1 -> Divide/1
  Divide1/1 -> Sum3/2
  Sum1/1 -> Divide1/1
  dT1/1 -> Gain1/1
  Gain1/1 -> Product/2
  Identity Matrix1/1 -> Sum/2
  Bus Selector1/1 -> Unit Delay Resettable External IC/3  "<signal1>"
  [reset] -> Unit Delay Resettable External IC/2
  Unit Delay Resettable External IC/1 -> Divide1/2, vel(k-1)/1
  initCon/1 -> Bus Selector1/1
  Bus Selector2/1 -> Sum5/1, Demux2/1  "<signal1>"
  Sum5/1 -> Switch1/3
  [reset] -> Switch1/2
  cor/1 -> Bus Selector2/1
  acc(k-1) from BODY to NAV/1(acc_Nav(k-1)) -> Unit Delay Resettable External IC1/1, Unit Delay Resettable External IC1/3
  Unit Delay Resettable External IC1/1 -> Sum2/4
  [reset] -> Unit Delay Resettable External IC1/2
  reset/1 -> [reset]
  Unit Delay External IC/1 -> Sum2/1
  Switch1/1 -> vel/1, Unit Delay Resettable External IC/1
  Demux2/1 -> corVel/1
  Demux2/2 -> corVel/2
  Demux2/3 -> corVel/3

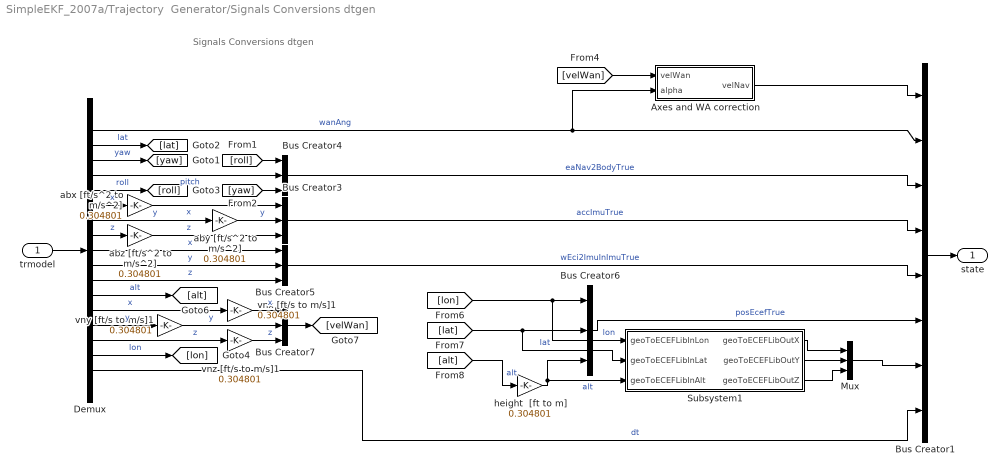
== system SimpleEKF_2007a/Trajectory  Generator/Signals Conversions dtgen ==
  note: Signals Conversions dtgen
  trmodel : Inport  OutDataType=fixdt(1,16,0)  OutScaling=[]
  Axes and WA correction : Subsystem
      settings: CopyFcn=|
      | if exist('gnlib_subsystem')
      |    gnlib_subsystem(gcbh, 'title')
      | end
      settings: NameChangeFcn=|
      | if exist('gnlib_subsystem')
      |    gnlib_subsystem(gcbh, 'title')
      | end
  Bus Creator1 : BusCreator  Inputs=8
  Bus Creator{3..7} (5 alike) : BusCreator  Inputs=3
  Demux : Demux  Outputs=17
  Mux : Mux  Inputs=3
  Subsystem1 : Subsystem
  "abx [ft/s^2 to m/s^2] " : Gain  Gain=0.304801  ParameterDataType=fixdt(1,16,0)  ParameterScaling=[]  OutDataType=fixdt(1,16,0)  OutScaling=[]
  aby [ft/s^2 to m/s^2] : Gain  Gain=0.304801  ParameterDataType=fixdt(1,16,0)  ParameterScaling=[]  OutDataType=fixdt(1,16,0)  OutScaling=[]
  abz [ft/s^2 to m/s^2] : Gain  Gain=0.304801  ParameterDataType=fixdt(1,16,0)  ParameterScaling=[]  OutDataType=fixdt(1,16,0)  OutScaling=[]
  height  [ft to m] : Gain  Gain=0.304801  ParameterDataType=fixdt(1,16,0)  ParameterScaling=[]  OutDataType=fixdt(1,16,0)  OutScaling=[]
  vnx [ft/s to m/s]1 : Gain  Gain=0.304801  ParameterDataType=fixdt(1,16,0)  ParameterScaling=[]  OutDataType=fixdt(1,16,0)  OutScaling=[]
  vny [ft/s to m/s]1 : Gain  Gain=0.304801  ParameterDataType=fixdt(1,16,0)  ParameterScaling=[]  OutDataType=fixdt(1,16,0)  OutScaling=[]
  vnz [ft/s to m/s]1 : Gain  Gain=0.304801  ParameterDataType=fixdt(1,16,0)  ParameterScaling=[]  OutDataType=fixdt(1,16,0)  OutScaling=[]
  state : Outport  OutDataType=fixdt(1,16,0)  OutScaling=[]
  wires:
  [yaw] -> Bus Creator4/3
  [roll] -> Bus Creator4/1
  Demux/5 -> [roll]  "roll"
  Demux/3 -> [yaw]  "yaw"
  Demux/17 -> Bus Creator1/8  "dt"
  Bus Creator5/1 -> Bus Creator1/5  "wEci2ImuInImuTrue"
  Bus Creator3/1 -> Bus Creator1/4  "accImuTrue"
  Axes and WA correction/1(velNav) -> Bus Creator1/1
  Demux/1 -> Axes and WA correction/2(alpha), Bus Creator1/2  "wanAng"
  [velWan] -> Axes and WA correction/1(velWan)
  [alt] -> height  [ft to m]/1  "alt"
  [lat] -> Bus Creator6/2, Subsystem1/2(geoToECEFLibInLat)  "lat"
  [lon] -> Bus Creator6/1, Subsystem1/1(geoToECEFLibInLon)  "lon"
  Demux/16 -> [lon]  "lon"
  Bus Creator4/1 -> Bus Creator1/3  "eaNav2BodyTrue"
  Bus Creator7/1 -> [velWan]
  vnz [ft/s to m/s]1/1 -> Bus Creator7/3  "z"
  vnx [ft/s to m/s]1/1 -> Bus Creator7/1  "x"
  vny [ft/s to m/s]1/1 -> Bus Creator7/2  "y"
  Demux/15 -> vnz [ft/s to m/s]1/1  "z"
  Demux/14 -> vny [ft/s to m/s]1/1  "y"
  Demux/13 -> vnx [ft/s to m/s]1/1  "x"
  Demux/12 -> [alt]  "alt"
  Demux/11 -> Bus Creator5/3  "z"
  Demux/10 -> Bus Creator5/2  "y"
  Demux/9 -> Bus Creator5/1  "x"
  Demux/2 -> [lat]  "lat"
  Demux/4 -> Bus Creator4/2  "pitch"
  Demux/8 -> abz [ft/s^2 to m/s^2]/1  "z"
  Demux/7 -> aby [ft/s^2 to m/s^2]/1  "y"
  Demux/6 -> "abx [ft/s^2 to m/s^2] "/1  "x"
  Bus Creator1/1 -> state/1
  trmodel/1 -> Demux/1
  Bus Creator6/1 -> Bus Creator1/6  "posEcefTrue"
  height  [ft to m]/1 -> Bus Creator6/3, Subsystem1/3(geoToECEFLibInAlt)  "alt"
  "abx [ft/s^2 to m/s^2] "/1 -> Bus Creator3/1  "x"
  aby [ft/s^2 to m/s^2]/1 -> Bus Creator3/2  "y"
  abz [ft/s^2 to m/s^2]/1 -> Bus Creator3/3  "z"
  Subsystem1/1(geoToECEFLibOutX) -> Mux/1
  Subsystem1/2(geoToECEFLibOutY) -> Mux/2
  Subsystem1/3(geoToECEFLibOutZ) -> Mux/3
  Mux/1 -> Bus Creator1/7

== system SimpleEKF_2007a/Trajectory  Generator/Signals Conversions trmodel ==
  note: Signals Conversions trmodel
  note: 1/delta time from dtgen
  note: ft/s^2 to m/s^2
  dtgen : Inport  OutDataType=fixdt(1,16,0)  OutScaling=[]
  Bus Creator1 : BusCreator  Inputs=2
  Bus Creator2 : BusCreator  Inputs=3
  Bus Creator3 : BusCreator  Inputs=3
  Demux : Demux  Outputs=6
  aby [ft/s^2 to m/s^2]{,1..5} (6 alike) : Gain  Gain=100  ParameterDataType=fixdt(1,16,0)  ParameterScaling=[]  OutDataType=fixdt(1,16,0)  OutScaling=[]
  vnx [ft/s to m/s] : Gain  Gain=0.304801  ParameterDataType=fixdt(1,16,0)  ParameterScaling=[]  OutDataType=fixdt(1,16,0)  OutScaling=[]
  vny [ft/s to m/s] : Gain  Gain=0.304801  ParameterDataType=fixdt(1,16,0)  ParameterScaling=[]  OutDataType=fixdt(1,16,0)  OutScaling=[]
  vnz [ft/s to m/s] : Gain  Gain=0.304801  ParameterDataType=fixdt(1,16,0)  ParameterScaling=[]  OutDataType=fixdt(1,16,0)  OutScaling=[]
  imu : Outport  OutDataType=fixdt(1,16,0)  OutScaling=[]
  wires:
  dtgen/1 -> Demux/1
  Bus Creator1/1 -> imu/1
  Demux/1 -> aby [ft/s^2 to m/s^2]/1  "x"
  Demux/2 -> aby [ft/s^2 to m/s^2]1/1  "y"
  Demux/3 -> aby [ft/s^2 to m/s^2]2/1  "z"
  Demux/4 -> aby [ft/s^2 to m/s^2]3/1  "x"
  Demux/5 -> aby [ft/s^2 to m/s^2]4/1  "y"
  Demux/6 -> aby [ft/s^2 to m/s^2]5/1  "z"
  aby [ft/s^2 to m/s^2]5/1 -> vnx [ft/s to m/s]/1  "z"
  aby [ft/s^2 to m/s^2]4/1 -> vnz [ft/s to m/s]/1  "y"
  aby [ft/s^2 to m/s^2]3/1 -> vny [ft/s to m/s]/1  "x"
  aby [ft/s^2 to m/s^2]2/1 -> Bus Creator3/3  "z"
  aby [ft/s^2 to m/s^2]1/1 -> Bus Creator3/2  "y"
  aby [ft/s^2 to m/s^2]/1 -> Bus Creator3/1  "x"
  vny [ft/s to m/s]/1 -> Bus Creator2/1  "x"
  vnz [ft/s to m/s]/1 -> Bus Creator2/2  "y"
  vnx [ft/s to m/s]/1 -> Bus Creator2/3  "z"
  Bus Creator3/1 -> Bus Creator1/1  "wEci2ImuInImuTrue"
  Bus Creator2/1 -> Bus Creator1/2  "accImuTrue"

== system SimpleEKF_2007a/Display results/Subsystem1/square ==
  squareLibIn : Inport  DataType=double  OutDataType=fixdt(1,16,0)  OutScaling=[]
  Product : Product  OutDataType=fixdt(1,16,0)  OutScaling=[]  RndMeth=Zero
  squareLibOut : Outport  OutDataType=fixdt(1,16,0)  OutScaling=[]  InitialOutput=0
  wires:
  squareLibIn/1 -> Product/2, Product/1
  Product/1 -> squareLibOut/1

== system SimpleEKF_2007a/Display results/Subsystem2/square ==
  squareLibIn : Inport  DataType=double  OutDataType=fixdt(1,16,0)  OutScaling=[]
  Product : Product  OutDataType=fixdt(1,16,0)  OutScaling=[]  RndMeth=Zero
  squareLibOut : Outport  OutDataType=fixdt(1,16,0)  OutScaling=[]  InitialOutput=0
  wires:
  squareLibIn/1 -> Product/2, Product/1
  Product/1 -> squareLibOut/1

== system SimpleEKF_2007a/EKF/MeasureVector/GPS ==
  posTrue : Inport  OutDataType=fixdt(1,16,0)  OutScaling=[]
  velTrue : Inport  Port=2  OutDataType=fixdt(1,16,0)  OutScaling=[]
  Add : Sum  OutDataType=fixdt(1,16,0)  OutScaling=[]
  Add1 : Sum  OutDataType=fixdt(1,16,0)  OutScaling=[]
  Demux1 : Demux  Outputs=3
  Demux3 : Demux  Outputs=3
  Demux4 : Demux  Outputs=3
  GPSposError : Scope  NumInputPorts=3
      settings: TimeRange=100  YMin=-7e+006~-1.1e+007~-1.1e+007  YMax=7e+006~2e+006~2e+006  SaveName=ScopeData3
  Mux : Mux  Inputs=3
  Mux1 : Mux  Inputs=3
  Random Number : RandomNumber  Variance=[1e-12 1e-12 2.5]  Seed=[55 45 60]  SampleTime=0.01
  Random Number1 : RandomNumber  Variance=0.01^2  Seed=[23 15 30]  SampleTime=0.01
  Subsystem1 : Subsystem
  Subsystem2 : Subsystem
  Sum2 : Sum  Inputs=+-  OutDataType=fixdt(1,16,0)  OutScaling=[]  SampleTime=0.01
  posGps : Outport  OutDataType=fixdt(1,16,0)  OutScaling=[]
  velGps : Outport  Port=2  OutDataType=fixdt(1,16,0)  OutScaling=[]
  wires:
  Random Number/1 -> Add/2
  Add/1 -> posGps/1, Demux1/1
  Random Number1/1 -> Add1/2
  Add1/1 -> velGps/1
  velTrue/1 -> Add1/1
  posTrue/1 -> Add/1, Demux3/1
  Demux1/1 -> Subsystem2/1(geoToECEFLibInLon)
  Demux1/2 -> Subsystem2/2(geoToECEFLibInLat)
  Demux1/3 -> Subsystem2/3(geoToECEFLibInAlt)
  Demux3/1 -> Subsystem1/1(geoToECEFLibInLon)
  Demux3/2 -> Subsystem1/2(geoToECEFLibInLat)
  Demux3/3 -> Subsystem1/3(geoToECEFLibInAlt)
  Sum2/1 -> Demux4/1
  Mux/1 -> Sum2/1
  Mux1/1 -> Sum2/2
  Demux4/1 -> GPSposError/1
  Demux4/2 -> GPSposError/2
  Demux4/3 -> GPSposError/3
  Subsystem2/1(geoToECEFLibOutX) -> Mux/1
  Subsystem2/2(geoToECEFLibOutY) -> Mux/2
  Subsystem2/3(geoToECEFLibOutZ) -> Mux/3
  Subsystem1/1(geoToECEFLibOutX) -> Mux1/1
  Subsystem1/2(geoToECEFLibOutY) -> Mux1/2
  Subsystem1/3(geoToECEFLibOutZ) -> Mux1/3
